simulink model "Explorer1632_LCD"  (Simulink 7.5)
settings: Solver=FixedStepDiscrete  StartTime=0.0  StopTime=200  FixedStep=0.001  RelTol=1e-3
undefined symbols (not defined in the file or in its folder): A0, B15, D4, Max, ms, Pin, Resol, us
libraries: MCHP_Blockset x17, simulink x5
settings Model: Creator=M17129  LastModifiedBy=Lubin Kerhuel
settings OptimizationCC: InlineParams=on  InlineInvariantSignals=on  EnhancedBackFolding=on  ExpressionDepthLimit=128  EfficientFloat2IntCast=on  OptimizeModelRefInitCode=on  LifeSpan=1
settings DebuggingCC: UnderspecifiedInitializationDetection=Simplified  MergeDetectMultiDrivingBlocksExec=error  SolverPrmCheckMsg=none  FcnCallInpInsideContextMsg=Enable All  StateNameClashWarn=none
settings HardwareCC: ProdBitPerInt=16  ProdIntDivRoundTo=Zero  ProdEndianess=LittleEndian  ProdWordSize=16  ProdHWDeviceType=Generic->Custom
settings ModelReferenceCC: ModelReferenceNumInstancesAllowed=Single
settings RTWCC: SystemTargetFile=MCHP_dsPIC_stf.tlc  TemplateMakefile=MCHP_dsPIC.tmf  Description=Microchip Embedded Target PIC24 dsPIC30 dsPIC33 (real-time)  GenerateReport=on  ProcessScript=MCHP_dsPIC_stf_make_rtw_hook  CustomInclude=./clib  CustomSource=Explorer1332_LCD_customCFile.c  IncludeHyperlinkInReport=on  GenerateTraceInfo=on  GenerateTraceReport=on  GenerateTraceReportSl=on  GenerateTraceReportSf=on  GenerateTraceReportEml=on
settings CodeAppCC: ForceParamTrailComments=on  IgnoreCustomStorageClasses=off  MaxIdLength=255  SimulinkDataObjDesc=on  SFDataObjDesc=on  CustomSymbolStrType=$N$R$M_T  InsertBlockDesc=on
settings STFCustomTargetCC: TargetLibSuffix=_lib.a  TargetFunctionLibrary=C89/C90 (ANSI)  IncludeMdlTerminateFcn=off  CombineOutputUpdateFcns=on  SuppressErrorStatus=on  ERTCustomFileBanners=on  SupportContinuousTime=off  SystemTargetFile=MCHP_dsPIC_stf.tlc
settings ERTTargetCC: TargetLibSuffix=_lib.a  TargetFunctionLibrary=C89/C90 (ANSI)  MultiwordLength=2048  ParMdlRefBuildCompliant=off  CompOptLevelCompliant=off  IncludeMdlTerminateFcn=off  SuppressErrorStatus=on  ERTFirstTimeCompliant=off  SupportNonInlinedSFcns=on  ModelStepFunctionPrototypeControlCompliant=off  CPPClassGenCompliant=off  ExtModeMexFile=ext_serial_win32_comm_no_acks  InlinedParameterPlacement=NonHierarchical  ERTSrcFileBannerTemplate=MCHP_dsPIC_code_template.cgt  ERTHdrFileBannerTemplate=MCHP_dsPIC_code_template.cgt  ERTDataSrcFileTemplate=MCHP_dsPIC_code_template.cgt  ERTDataHdrFileTemplate=MCHP_dsPIC_code_template.cgt  ERTCustomFileTemplate=MCHP_main.tlc
settings CustomProperty: DataType=string  Value=33EP512MU810
settings EnumStrPairs: String=elf

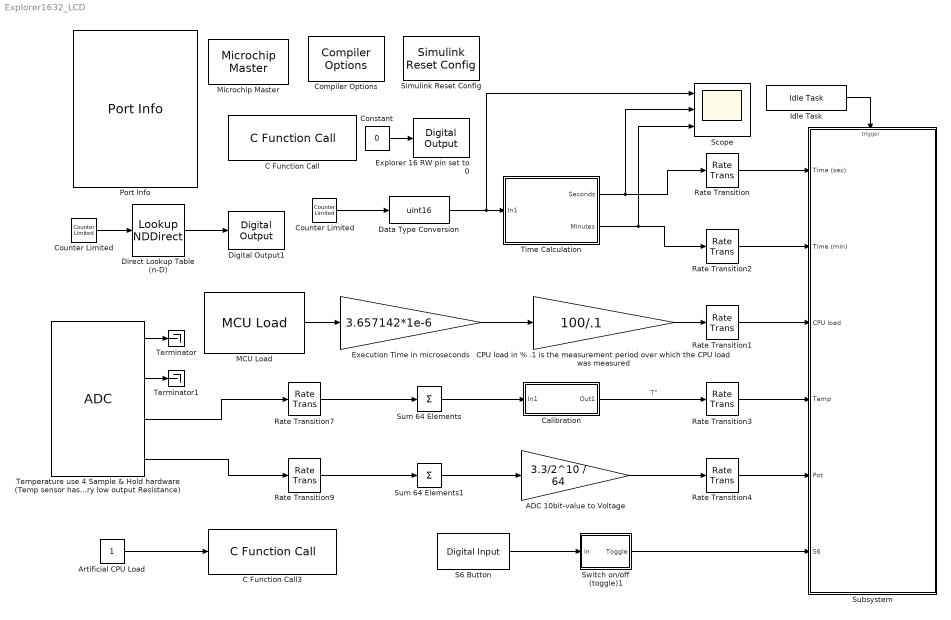
== system Explorer1632_LCD ==
  ADC 10bit-value to Voltage : Gain  Gain=3.3/2^10 / 64  OutDataTypeMode=double  OutDataTypeStr=double
  Artificial CPU Load : Constant  OutDataTypeStr=Inherit: Inherit via back propagation
  C Function Call : MCHP_Blockset/User Functions/C Function Call  ParseFilesChkbx=on  ListFunctions1=Custom Function  Function1=void LCD_StartUp()  AddHeaderDeclaration=off  Function1Type=only once at power-up time  FctReturnBlockOut=off  DataCollected="s.chksm={ '168203-Apr-2017 17:13:43'};s.File1=reshape({ '  void  LCD_StartUp()','  void  PrintMinutes(unsigned int minutes)','  void  PrintSeconds(unsigned int seconds)','  void  PrintVoltage(double v)','  void  PrintTemperature(double temp)','  void  PrintCPU(double CPU_Load)'},1,6);"  ORDERING=None  SampleTime=1  S_INPUT=[]  S_INPUT_Size=[]  S_OUTPUT=[]  S_OUTPUT_Size=[]  S_ListCustomDatatype=S.S_ListCustomDatatype={};  MCHP_CRC=1481661  MCHP_MASTERLINK=Explorer1632_LCD/Microchip Master  PinDigitalInput=[]  PinDigitalOutput=[B15 D4 E[4:7]]  PinAnalogInput=[]  MCHP_PORT={C Function LCD_StartUp}{CFct}10:1:B15;{C Function LCD_StartUp}{CFct}10:1:D4;{C Function LCD_StartUp}{CFct}10:1:E4;{C Function LCD_StartUp}{CFct}10:1:E5;{C Function LCD_StartUp}{CFct}10:1:E6;{C Function LCD_StartUp}{CFct}10:1:E7;
  C Function Call3 : MCHP_Blockset/User Functions/C Function Call  ParseFilesChkbx=off  ListFunctions1=Custom Function  Function1=extern void __delay_us(unsigned long t_us);  AddHeaderDeclaration=off  Function1Type=when block is updated (default)  Fct1BlockIn=t_us  FctReturnBlockOut=off  DataCollected=0  ORDERING=None  SampleTime=.001  S_INPUT=[7]  S_INPUT_Size="[0  0  0  0  0  0  0  0  0  0]"  S_OUTPUT=[]  S_OUTPUT_Size=[]  S_ListCustomDatatype=S.S_ListCustomDatatype={};  MCHP_CRC=972831  MCHP_MASTERLINK=Explorer1632_LCD/Microchip Master  PinDigitalInput=[]  PinDigitalOutput=[]  PinAnalogInput=[]
  CPU load in % .1 is the measurement period over which the CPU load was measured : Gain  Gain=100/.1  ParamDataTypeStr=Inherit: Inherit from 'Gain'  OutDataTypeMode=double  OutDataTypeStr=double
  "Calibration " : Subsystem
  Compiler Options : MCHP_Blockset/System Configuration/Compiler Options  Priority=1  LATEST_CMPLR=on  COMP_LIST=Dynamic Options  COMP_LIST_TXT=xc16 - v1.36  USE_64BIT_DOUBLE=off  MCHP_MULTITHREAD_COMPILATION=on  UseCustom_LinkerScript=off  MCHP_MASTERLINK=Explorer1632_LCD/Microchip Master  OPTIMIZATION_LEVEL=1  OPTIMIZATION_FLTO=on  OPTIMIZATION_REORDER=off  UNROLL_LOOPS=on  PROCEDURAL_ABSTRACTION=off  MPLAB_LINKLIB=default  MPLAB_LINKLIB1=default  MCODE=is less than 32768 (faster)  MCONST=in data memory  MDATA=Use only memory below address 8192 (faster)  MSCALAR=Use only memory below address 8192 (faster)  MLARGEARRAY=off  MAGGREGATE=off  HEAP_SIZE=0  OMF=elf  DEBUG_INFO=off  ProduceHexOutput=off  AssemblyListing=off  NO_EDS_WARN=on  PRINT_STATISTICS=off
  Constant : Constant  Value=0  OutDataType=fixdt(1, 16)  OutScaling=2^0  OutDataTypeStr=Inherit: Inherit via back propagation
  Counter Limited : simulink/Sources/Counter Limited  SystemSampleTime=-1  uplimit=59  tsamp=1
  "Counter Limited " : simulink/Sources/Counter Limited  SystemSampleTime=-1  uplimit=11  tsamp=.08
  Data Type Conversion : DataTypeConversion  OutDataTypeMode=uint16  OutDataTypeStr=uint16  ConvertRealWorld=Stored Integer (SI)
  Digital Output1 : MCHP_Blockset/Digital IO/Digital Output  SystemSampleTime=-1  PORT=Dynamic Options  PORT_TXT="A   [ 0  1  2  3  4  5  6  7  9  10  14  15 ]"  PIN=[1:7]  PACK=on  SIMULTANEOUS=off  READPREVIOUS=off  ORDERING=None  SampleTime=-1  MCHP_MASTERLINK=Explorer1632_LCD/Microchip Master
  Direct Lookup Table (n-D) : LookupNDDirect  NumberOfTableDimensions=1  Table=[ 2 4 8 16 32 64 128 64 32 16 8 4 ]  TableDataTypeStr=uint16
  Execution Time in microseconds : Gain  Gain=3.657142*1e-6  ParamDataTypeStr=Inherit: Inherit from 'Gain'  OutDataTypeMode=double  OutDataTypeStr=double
  Explorer 16 RW pin set to 0 : MCHP_Blockset/Digital IO/Digital Output  SystemSampleTime=-1  PORT=Dynamic Options  PORT_TXT="D   [ 0 : 15 ]"  PIN=5  PACK=off  SIMULTANEOUS=off  READPREVIOUS=off  ORDERING=None  SampleTime=inf  MCHP_MASTERLINK=Explorer1632_LCD/Microchip Master
  Idle Task : MCHP_Blockset/System Functions/Idle Task  MCHP_MASTERLINK=Explorer1632_LCD/Microchip Master
  MCU Load : MCHP_Blockset/Profiling/MCU Load  MCULoadPin=Dynamic Options  MCULoadPin_TXT=None  MCULoadMeasure=on  TIMER_Resolution=Dynamic Options  TIMER_Resolution_TXT="Resol: 3.657(us)  -  Max: 240(ms)"  MCHP_TIMER_REQUEST={MCU_Load}{MCU_Load}21:5:0:0:[]:16777216;  MCHP_TIMER_RESULT=[1 65535 ]  MCHP_MASTERLINK=Explorer1632_LCD/Microchip Master  MCHP_COMPILED_INFO="CompiledSampleTime= [0.10000000000000001   0 ];CompiledInportDataTypes=[ ];CompiledInportDataWidth=[];"  Info="Timer 1:  Resol: 3.657142857(us)  -  Max: 239.675(ms)"  SampleTime=.1
  Microchip Master : MCHP_Blockset/System Configuration/Microchip Master  Priority=1  PICREF=33EP512MU810  TIMESTEP_REF="ADC  ( 0.001s + [0.11429%] ==> 0.0010011s )"  BUSYFLAG=Dynamic Options  BUSYFLAG_TXT=A0 / Pin[17]  PWRTEN=Not used  BOREN=Disable  BODENV=2.7V  BORV=Not used  FPWRT=128ms  DSBOREN=Enable ZPBOR during Deep Sleep Mode  DSLPBOR=Not used  MCLRE=Enabled  SMCLR=MCLR pin generates a normal system Reset  PMDL1WAY=Allow only one reconfiguration  RSTPRI=Device will obtain reset instruction from Primary flash  TEMP=Not used  SOSCSRC=Not used  SOSCSEL=Not used  IOL1WAY=Allow only one reconfiguration  ALTVREF=Not used  DISUVREG=Not used  DSSWEN=Not used  LPCFG=Not used  RTCBAT=Not used  VBTBOR=Not used  WUTSEL=Not used  POWERSAVE=off  FNOSC=Primary Oscillator (XT; HS; EC)  FPR=ECIO w/ PLL 16x  FOSFPR=HS3 w/PLL 16x  FOS=Internal Fast RC  FRANGE=High Range  OSCILLATOR_SELECT=Crystal / Ceramic resonator  OSCILLATOR_SELECT_spd=Crystal / Ceramic resonator  QUARTZ=8e+06  QUARTZ_spd=8e+06  POSCGAIN=2x gain setting  POSCBOOST=Boost the kick start of the oscillator  SOSCGAIN=2x gain setting  SOSCBOOST=Boost the kick start of the oscillator  ACTIV_PLL=on  ACTIV_PLL_spd=on  MIPS_DESIRED=70e+06  MIPS_DESIRED_spd=70e+06  FPLLMUL=Not used  FPLLIDIV=8x Divider  POSCFREQ=Not used  POSCMD=XT Crystal Oscillator Mode  POSCMOD=Primary Oscillator Disabled  MIPS=70 * 1e6  ACLKCON=Optimized for PWM resolution & ADC conversion speed  FPLLODIV=32x Divider  PLLKEN=Clock switch to PLL source will wait until the PLL lock signal is valid.  FCKSM=Clock switching is enabled;Fail-safe Clock Monitor is disabled  FCKSMEN=Sw Disabled; Mon Disabled  IESO=Disable  DSWDTPS=1:2^36  FWDTEN=Disable  FWDTWINSZ=Window size is 25%  FWPSA=1:512  FWPSA0=1:128  FWPSB=1:16  WDT=Disable  WDTPOST=1:32768  WDTPRE=1:128  WDTPS=1:32768  WINDIS=Watchdog Timer in Non-Window mode  WWDTEN=Non-Window mode  DSWDTEN=Enable DSWDT during Deep Sleep Mode  DSWDTOSC=Select LPRC as DSWDT Reference clock  FPBDIV=Not used  FSOSCEN=Enable SOSC  LPRCSEL=Not used  OSCIOFCN=Not used  OSCIOFNC=general purpose digital I/O pin  LVRCFG=Not used  PLL_96MHZ=Not used  PLL96MHZ=Not used  PLLDIV=Not used  WDTCLK=Not used  WDTCMX=Not used  WDTWIN=WDT Window is 25% of WDT period  XTCFG=24-32 MHz crystals  XTBST=Boost the kick-start  APL=Aux Flash Code protect is disabled  APLK=Aux Flash Write Protection and Code Protection is Disabled  AWRP=Auxiliary program memory is not write-protected  BSS=No Boot program Flash segment  BWP=Not used  BWRP=Boot Segment may be written  CP=Protection Disabled  EBS=No Boot EEPROM  ESS=No Segment Data EEPROM  GCP=Disable  GSS=General Segment Code protect is Disabled  GSS0=Not used  GSSK=General Segment Write Protection and Code Protection is Disabled  GWRP=General Segment may be written  PWP=Not used  RBS=No Boot RAM  RSS=No Secure RAM  SSS=No Secure Segment  SWRP=Secure segment may be written  WPCFG=Not used  WPDIS=Not used  WPEND=Not used  WPFP=Not used  ICESEL=Communicate on PGEC1/PGED1  ICS=Communicate on PGEC1 and PGED1  JTAGEN=Disable  COE=Not used  RES=Not used  DEBUG=Debugger is disabled  BACKBUG=Not used  BKBUG=Not used  ALTI2C=I2C mapped to SDA1/SCL1 pins  ALTI2C1=SDA1/SCK1 pins are selected as the I/O pins for I2C1  ALTI2C2=SDA2/SCK2 pins are selected as the I/O pins for I2C2  ALTI2C3=I2C3 mapped to SDA3/SCL3 pins  ALTQIO=QEA1; QEB1; INDX1 are selected as inputs to QEI1  ALTSS1=SS1A is selected as the I/O pin for SPI1  CMPPOL0=Hysteresis is applied to falling edge  CMPPOL1=Hysteresis is applied to falling edge  FCANIO=Not used  FETHIO=Default Ethernet I/O  FMIIEN=MII Enabled  FSRSSEL=Not used  FUSBIDIO=Controlled by the USB Module  FVBUSONIO=Not used  HPOL=Active High  HYST0=45 mV Hysteresis  HYST1=45 mV Hysteresis  I2C1SEL=Not used  LPOL=Active High  PWMPIN=Control with PORT/TRIS regs  RTCOSC=Not used  UPLLEN=USB PLL Disabled  UPLLIDIV=Not used  ATMOD8=Not used  ALTPMP=Not used  I2C2SEL=Not used  ALTADREF=Not used  ALTCVREF=Not used  PWMLOCK=PWM registers may be written without key sequence  INT_PRIORITY_DMA=0  MCHP_TIMER_RESULT=[ ]  MCHP_PORT={Busy Flag}{Busy}0:1:A0;  MCHP_PLLRegisters="[5    243  16385     -1     -1]"  MCHPVAR=MCHP.fcy.MIPS=70000000;MCHP.fcy.SYSCLK=70000000;MCHP.fcy.ADC=70000000;MCHP.fcy.Comparator=70000000;MCHP.fcy.I2C=70000000;MCHP.fcy.SPI=70000000;MCHP.fcy.UART=70000000;MCHP.fcy.Timers=70000000;MCHP.fcy.OC=70000000;MCHP.fcy.IC=70000000;MCHP.fcy.Ports=70000000;MCHP.fcy.QEI=70000000;MCHP.PowerSave=0;MCHP.TimeStepFactor=MCHP_Fun.Hex2num('3FF004AE5F60D755');MCHP.TimeStep_Timer=-1;MCHP.NTIMERS=9;MCHP.id.name='33EP512MU810';MCHP.id.N=reshape([33 512 810],1,3);MCHP.id.L=reshape({ 'EP','MU',''},1,3);MCHP.id.Arch=3;MCHP.periph.PPS.reg_RPINRx=reshape([-1 1 1 1 1 -1 1 1 1 1 1 1 1 1 1 1 1 1 1 1 1 1 -1 -1 1 1 1 1 1 1 1 1 1 1 1 1 1 1 1 1 1 1 1 -1 -1 -1 1 -1 -1 -1 -1 -1 1 1 1 1 1 1 1 1 1 -1 1 1 1 -1 1 1 1 1 1 1 1 1 -1 1 1 1 1 1 1 1 1 -1 1 1 1],1,87);MCHP.PPS.dsPIC.RP=reshape([-1 -1 -1 -1 -1 -1 -1 -1 -1 -1 -1 -1 -1 -1 -1 -1 -1 -1 -1 -1 -1 -1 -1 -1 -1 -1 -1 -1 -1 -1 -1 -1 -1 -1 -1 -1 -1 -1 -1 -1 -1 -1 -1 -1 -1 -1 -1 -1 -1 -1 -1 -1 -1 -1 -1 -1 -1 -1 -1 -1 -1 -1 -1 -1 48 49 50 51 52 53 54 55 -1 -1 -1 -1 -1 -1 -1 63 64 -1 66 -1 68 69 -1 71 -1 -1 -1 -1 -1 -1 -1 -1 80 81 82 83 84 85 -1 -1 88 -1 -1 -1 92 93 -1 -1 96 97 -1 -1 -1 -1 102 -1 104 -1 -1 -1 -1 109 110 111],1,128);MCHP.PPS.dsPIC.RPI=reshape([-1 -1 -1 -1 -1 -1 -1 -1 -1 -1 -1 -1 -1 -1 -1 -1 0 1 2 3 4 5 6 7 -1 -1 -1 -1 -1 -1 14 15 16 17 18 19 20 21 22 23 24 25 26 27 28 29 30 31 -1 33 34 35 36 -1 -1 -1 -1 -1 -1 -1 44 45 46 -1 -1 -1 -1 -1 -1 -1 -1 -1 56 57 58 59 60 61 62 -1 -1 65 -1 67 -1 -1 70 -1 72 73 -1 -1 -1 -1 -1 -1 -1 -1 -1 -1 -1 -1 -1 -1 -1 -1 -1 -1 -1 -1 -1 -1 -1 -1 -1 -1 -1 -1 -1 103 -1 105 -1 -1 108],1,125);MCHP.PPS.dsPIC.RPINR_list=reshape({ '1','INT1','INT2','INT3','INT4','T1CK','T2CK','T3CK','T4CK','T5CK','T6CK','T7CK','T8CK','T9CK','IC1','IC2','IC3','IC4','IC5','IC6','IC7','IC8','OCFA','OCFB','FLT1','FLT2','FLT3','FLT4','QEIA1','QEIB1','QEINDX1','QEIHOM1','QEIA2','QEIB2','QEINDX2','QEIHOM2','U1RX','U1CTS','U2RX','U2CTS','SDI1','SCK1_in','SS1_in','44','SDI2','SCK2_in','SS2_in','48','CSDIR','CSCK','COFS','52','C1RX','C2RX','U3RX','U3CTS','U4RX','U4CTS','SDI3','SCK3_in','SS3_in','62','SDI4','SCK4_in','SS4_in','66','IC9','IC10','IC11','IC12','IC13','IC14','IC15','IC16','OCFC','SYNCI1','SYNCI2','DTCMP1','DTCMP2','DTCMP3','DTCMP4','DTCMP5','DTCMP6','DTCMP7','FLT5','FLT6','FLT7','FLT8','89','SENT1','SENT2','92'},1,92);MCHP.PPS.dsPIC.RPOR_list=reshape({ '1','U1TX','U1RTS','U2TX','U2RTS','SDO1','SCK1_out','SS1_out','SDO2','SCK2_out','SS2_out','CSDO','CSCK','COFS','C1TX','C2TX','OC1','OC2','OC3','OC4','OC5','OC6','OC7','OC8','C1OUT','C2OUT','C3OUT','U3TX','U3RTS','U4TX','U4RTS','SDO3','SCK3_out','SS3_out','SDO4','SCK4_out','SS4_out','OC9','OC10','OC11','OC12','OC13','OC14','OC15','OC16','SYNCO1','SYNCO2','QEI1CCMP','QEI2CCMP','REFCLK','C4OUT','C5OUT','52','53','54','55','56','SENT1','SENT2'},1,59);MCHP.PPS.map_RPnR_RPORx=reshape([64 65 66 67 68 69 70 71 79 80 82 84 85 87 96 97 98 99 100 101 -1 -1 104 108 109 112 113 118 120 125 126 127],1,32);MCHP.Rx=reshape([17 25 -1 72 93 87 90 -1 -1 -1 -1 38 24 6 76 94 88 89 -1 -1 -1 -1 58 23 7 77 98 52 57 -1 -1 -1 -1 59 22 8 78 99 51 56 -1 -1 -1 -1 60 21 9 81 100 49 -1 -1 -1 -1 -1 61 20 -1 82 3 50 -1 -1 -1 -1 -1 91 26 -1 83 4 -1 10 -1 -1 -1 -1 92 27 -1 84 5 -1 11 -1 -1 -1 -1 -1 32 -1 68 18 53 12 -1 -1 -1 -1 28 33 -1 69 19 -1 14 -1 -1 -1 -1 29 34 -1 70 -1 -1 -1 -1 -1 -1 -1 -1 35 -1 71 -1 -1 -1 -1 -1 -1 -1 -1 41 63 79 -1 40 96 -1 -1 -1 -1 -1 42 73 80 -1 39 97 -1 -1 -1 -1 66 43 74 47 -1 -1 95 -1 -1 -1 -1 67 44 64 48 -1 -1 1 -1 -1 -1 -1],11,16);MCHP.ADC.ANtype=reshape([3 1],1,2);MCHP.ADC.ADCONx=reshape([47103 59391 40959 263 0 0],1,6);MCHP.ADC.ADCHS_0=reshape([40863 1799],1,2);MCHP.ADC.Flags=reshape([1 0],1,2);MCHP.ADC.Buffer=reshape([16 16],1,2);MCHP.ADC.port=reshape([16 17 18 19 20 21 22 23 24 25 26 27 28 29 30 31 33 34 35 36 72 73 6 7 64 65 66 67 68 69 70 71 -1 -1 -1 -1 -1 -1 -1 -1 -1 -1 -1 -1 -1 -1 -1 -1 -1 -1 -1 -1 -1 -1 -1 -1 -1],1,57);MCHP.ADC.port_ALT=reshape([-1 -1 -1 -1],1,4);MCHP.ADC.port_VrefP=10;MCHP.ADC.port_VrefM=9;MCHP.ADC.port_AVdd=-1;MCHP.ADC.port_AVss=-1;MCHP.ADC.ADCDATA=reshape([0 0 0 0 0 0 0 0 0 0 0 0 0 0 0 0 0 0 0 0 0 0 0 0 0 0 0 0 0 0 0 0 0 0 0 0 0 0 0 0 0 0 0 0 0 0 0 0 0 0 0 0 0 0 0 0 0],1,57);MCHP.ADC.HS_SAR.TRGSRC=reshape([0 0 0 0 0 0 0 0 0 0 0 0 0 0 0 0 0 0 0 0 0 0 0 0 0 0],1,26);MCHP.ADC.HS_SAR.nFilters=0;MCHP.ADC.HS_SAR.nDedicatedCore=0;MCHP.ADC.HS_SAR.CALIBRATION=0;MCHP.ADC.HS_SAR.ADCON1L=-1;MCHP.memory.RAM=53248;MCHP.memory.RAM_XBegin=4096;MCHP.memory.RAM_YBegin=36864;MCHP.memory.RAM_dma=reshape([53248 57344],1,2);MCHP.memory.FLASH_ECC=0;MCHP.DMA.Num=15;MCHP.DMA.CNTmax=16383;MCHP.QEI.QEICONx=reshape([49023 49023 -1 -1 -1 -1],1,6);MCHP.QEI.QEItype=2;MCHP.QEI.Port_QEI_INDX=reshape([-1 -1],1,2);MCHP.QEI.Port_QEI_QEA=reshape([-1 -1],1,2);MCHP.QEI.Port_QEI_QEB=reshape([-1 -1],1,2);MCHP.QEI.Port_QEI_UPDN=reshape([-1 -1],1,2);MCHP.INT.Port=reshape([48 32767 32767 32767 32767],1,5);MCHP.PWM_HS.Flags=reshape([6 2 1],1,3);MCHP.PWM.port_FLT=reshape([-1 -1 -1 -1 -1 -1 -1 -1 -1 -1 -1 -1 -1 -1 -1 -1 -1 -1 -1 -1 -1 -1 -1 -1 -1 -1 -1 -1 -1 -1 -1 -1 -1],1,33);MCHP.PWM.PWMRef=-1;MCHP.PWM.Flag=0;MCHP.PWM.Port_PWM_l=reshape([64 -1 66 -1 68 -1 70 -1 33 -1 35 -1 -1 -1 -1 -1 -1 -1 -1 -1 -1 -1 -1 -1],2,12);MCHP.PWM.Port_PWM_h=reshape([65 -1 67 -1 69 -1 71 -1 34 -1 36 -1 -1 -1 -1 -1 -1 -1 -1 -1 -1 -1 -1 -1],2,12);MCHP.PWM_HS_FEP.nEVTOUT=-1;MCHP.IC.Port=reshape([32767 32767 32767 32767 32767 32767 32767 32767 32767 32767 32767 32767 32767 32767 32767 32767],1,16);MCHP.IC.type=1;MCHP.OC.Port=reshape([32767 32767 32767 32767 32767 32767 32767 32767 32767 32767 32767 32767 32767 32767 32767 32767],1,16);MCHP.OC.type=1;MCHP.CN.Port=reshape([-1 -1 -1 -1 -1 -1 -1 -1 -1 -1 -1 -1 -1 -1 -1 -1 -1 -1 -1 -1 -1 -1 -1 -1 -1 -1 -1 -1 -1 -1 -1 -1 -1 -1 -1 -1 -1 -1 -1 -1 -1 -1 -1 -1 -1 -1 -1 -1 -1 -1 -1 -1 -1 -1 -1 -1 -1 -1 -1 -1 -1 -1 -1 -1 -1 -1 -1 -1 -1 -1 -1 -1 -1 -1 -1 -1 -1 -1 -1 -1 -1 -1 -1 -1 -1],1,85);MCHP.CN.PullUp=reshape([50943 65535 61470 65535 1023 12607 62403 0 0 0 0],1,11);MCHP.CN.type=1;MCHP.CN.Flag_PullDown=1;MCHP.SPI.Refs=reshape([1 2 3 4 0 0],1,6);MCHP.SPI.SPIxCON1=8191;MCHP.SPI.SPIxCON2=57347;MCHP.SPI.Port_SDI=reshape([-1 103 -1 -1 -1 -1],1,6);MCHP.SPI.Port_SDO=reshape([-1 104 -1 -1 -1 -1],1,6);MCHP.SPI.Port_SCK=reshape([-1 102 -1 -1 -1 -1],1,6);MCHP.SPI.Port_SS=reshape([-1 -1 -1 -1 -1 -1],1,6);MCHP.I2C.Refs=reshape([1 2 0 0 0],1,5);MCHP.I2C.I2CxCON=49151;MCHP.I2C.NewRegName=1;MCHP.I2C.Port_SDA=reshape([-1 84 -1 -1 -1],1,5);MCHP.I2C.Port_SCL=reshape([-1 85 -1 -1 -1],1,5);MCHP.I2C.Port_ASDA=reshape([57 3 -1 -1 -1],1,5);MCHP.I2C.Port_ASCL=reshape([58 2 -1 -1 -1],1,5);MCHP.I2C.Fuse_Port_SCL_SDA=reshape([17 1 18 1 -1 -1 -1 -1 -1 -1],2,5);MCHP.I2C.Fuse_Port_ASCL_ASDA=reshape([17 2 18 2 -1 -1 -1 -1 -1 -1],2,5);MCHP.SCCP.nSCCP=0;MCHP.SCCP.MCCP=reshape([0 0 0 0 0 0 0 0 0],1,9);MCHP.PGA.Port_PGA1P=reshape([-1 -1 -1 -1],1,4);MCHP.PGA.Port_PGA1N=reshape([-1 -1 -1 -1],1,4);MCHP.PGA.Port_PGA2P=reshape([-1 -1 -1 -1],1,4);MCHP.PGA.Port_PGA2N=reshape([-1 -1 -1 -1],1,4);MCHP.PGA.Num=0;MCHP.HS_AnalogComparator.Port_CMP1=reshape([-1 -1 -1 -1],1,4);MCHP.HS_AnalogComparator.Port_CMP2=reshape([-1 -1 -1 -1],1,4);MCHP.HS_AnalogComparator.Port_CMP3=reshape([-1 -1 -1 -1],1,4);MCHP.HS_AnalogComparator.Port_CMP4=reshape([-1 -1 -1 -1],1,4);MCHP.HS_AnalogComparator.PORT_EXTREFx=reshape([-1 -1],1,2);MCHP.HS_AnalogComparator.Port_DACOUTx=reshape([-1 -1],1,2);MCHP.HS_AnalogComparator.Num=0;MCHP.Comp.Port_CVrefin=-1;MCHP.Comp.Port_CVref=26;MCHP.Comp.Port_CVref1O=-1;MCHP.Comp.Port_CVref2O=-1;MCHP.Comp.Port_CxOUT=reshape([32767 32767 32767 -1 -1],1,5);MCHP.Comp.Port_OAxOUT=reshape([-1 -1 -1 -1 -1],1,5);MCHP.Comp.Port_CxINP=reshape([21 19 55 -1 -1],1,5);MCHP.Comp.Port_CxINM=reshape([103 20 102 -1 105 18 104 -1 46 54 45 -1 -1 -1 -1 -1 -1 -1 -1 -1],4,5);MCHP.Comp.Port_OAxINP=reshape([-1 -1 -1 -1 -1],1,5);MCHP.Comp.Port_OAxINM=reshape([-1 -1 -1 -1 -1],1,5);MCHP.Comp.nComp=reshape([3 0 0],1,3);MCHP.Comp.OpAmp=0;MCHP.Comp.CVRCON=reshape([2047 0],1,2);MCHP.CDAC.Port_DACx=reshape([-1 -1 -1],1,3);MCHP.CDAC.nCDAC=0;MCHP.UART.port_Rx=reshape([32767 32767 32767 32767 -1 -1],1,6);MCHP.UART.port_Tx=reshape([32767 32767 32767 32767 -1 -1],1,6);MCHP.UART.port_ARx=reshape([-1 -1],1,2);MCHP.UART.port_ATx=reshape([-1 -1],1,2);MCHP.UART.port_RTS=reshape([32767 32767 32767 32767 -1 -1],1,6);MCHP.UART.port_CTS=reshape([32767 32767 32767 32767 -1 -1],1,6);MCHP.UART.reg_UxMODE=reshape([48127 48127 48127 48127 -1 -1],1,6);MCHP.UART.reg_UxSTA=reshape([61439 61439 61439 61439 -1 -1],1,6);MCHP.modsrc.DOS_02551_cpu_16bit_v7=0;MCHP.modsrc.DOS_01520_wdt_dmt_upb_v1_16bit=0;MCHP.modsrc.DOS_02359a_sent_j2716_upb_v1=0;MCHP.modsrc.DOS_02672_math_progcrc_upb_v1_16bit=0;MCHP.modsrc.DOS_01577_cla_clc_upb_v1=0;MCHP.modsrc.DOS_02915_ecc_v2=0;MCHP.modsrc.DOS_02673_tmr_classa_upb_v1_16bit=0;MCHP.modsrc.DOS_01494_qei_32b_upb_v1_16bit=0;MCHP.modsrc.DOS_02552_msi_upb_v1_Master=0;MCHP.modsrc.DOS_01441_i2c_upb_v1_16bit_TLAH=0;MCHP.modsrc.DOS_03076_uart_protocol_upb_v1_16bit=0;MCHP.modsrc.DOS_01482=0;MCHP.modsrc.DOS_01483_pwm_16bit=0;MCHP.modsrc.DOS_03247_CAN_FD_UPB_V2_16_bit=0;MCHP.modsrc.DOS_02497_WACV=0;MCHP.modsrc.DOS_02316_nvm_ctrl_v1_16bit=0;MCHP.modsrc.DOS_02653_afe_current_bias_ctrl_upb_v1_16bit=0;MCHP.modsrc.DOS_01459_ptg_pc_upb_v1_16bit=0;MCHP.modsrc.DOS_01512_ccp_mccp_upb_v1_16bit=0;MCHP.modsrc.DOS_02519_dma_sfr_16bit_v2=0;MCHP.modsrc.DOS_02508c11=0;MCHP.modsrc.DOS_02475_dac_pdm_nbit_upb_v1_16bit=0;MCHP.modsrc.DOS_02467_gpio_upb_v1_16bit=0;MCHP.modsrc.DOS_00805_rst_integration_v4=0;MCHP.modsrc.DOS_02659_clk_sib_v12=0;MCHP.modsrc.DOS_02674_wdt_upb_v1_16bit=0;MCHP.modsrc.DOS_01407=0;MCHP.modsrc.DOS_02552_msi_upb_v1_Slave=0;MCHP.modsrc.DOS_02593_amp_pga_ctrl_pb_v2_16bit=0;MCHP.modsrc.DOS_01461_afe_ctmu_con_upb_v1_16bit=0;MCHP.modsrc.DOS_02497_WACA=0;MCHP.modsrc.DOS_02478_uart_irda_upb_v1_16bit=0;MCHP.modsrc.DOS_00929=1;MCHP.modsrc.DOS_01198=1;MCHP.modsrc.DOS_03029_WACH=0;MCHP.modsrc.DOS_02472_ppi_pmp16_upb_v1_16bit=0;MCHP.modsrc.DOS_02949_WACG=0;MCHP.modsrc.DOS_03349_amp_pad_opamp_ctrl_upb_v1=0;MCHP.modsrc.DOS_02237_osc_dco_ctrl_upb_v1_16bit=0;MCHP.modsrc.DOS_03662_WACU=0;MCHP.modsrc.DOS_03994_WAC07_Module=0;MCHP.modsrc.DOS_00794=1;MCHP.modsrc.DOS_00931=1;MCHP.modsrc.DOS_00932=1;MCHP.modsrc.DOS_00942=1;MCHP.modsrc.DOS_00938=1;MCHP.modsrc.DOS_00996=1;MCHP.modsrc.DOS_00997=1;MCHP.modsrc.DOS_00998=1;MCHP.modsrc.DOS_00209=1;MCHP.modsrc.DOS_01555_adc=0;MCHP.modsrc.DOS_01293=0;MCHP.modsrc.DOS_00828=1;MCHP.modsrc.DOS_01116=1;MCHP.modsrc.DOS_01017_RPORx=1;MCHP.modsrc.DOS_01017_RPINRx=1;MCHP.modsrc.DOS_01555_nvm_tsmc18_v2_16bit=0;MCHP.modsrc.DOS_00804=1;MCHP.modsrc.DOS_00826=1;MCHP.modsrc.DOS_01555_TLAK_PMDx=0;MCHP.modsrc.DOS_01555_TLAK_INT_=0;MCHP.modsrc.DOS_00933=1;MCHP.modsrc.DOS_01555=0;MCHP.modsrc.DOS_01555_ptg=0;MCHP.modsrc.DOS_00958=1;MCHP.modsrc.DOS_01117_PORTx=1;MCHP.modsrc.DOS_00999=1;MCHP.modsrc.DOS_01041=1;MCHP.modsrc.DOS_00892=1;MCHP.modsrc.DOS_01287_TLAC_PMDx=0;MCHP.modsrc.DOS_01287_TLAC_INT_=0;MCHP.modsrc.DOS_01424=0;MCHP.modsrc.DOS_01332=0;MCHP.modsrc.DOS_01468_PMBA_current_source=0;MCHP.modsrc.DOS_02291_PGA=0;MCHP.modsrc.DOS_01467_Comparator=0;MCHP.modsrc.DOS_01498_TLAY=0;MCHP.modsrc.DOS_00993_PLL_120MHz=0;MCHP.modsrc.DOS_01332_ptg_pc_v1=0;MCHP.modsrc.DOS_00958_pwm_TLAY=0;MCHP.modsrc.TLAY_IOPorts=0;MCHP.modsrc.DOS_00929q=0;MCHP.modsrc.DOS_02415_spi_v5=0;MCHP.modsrc.DOS_RPINRx_16bit_2=0;MCHP.modsrc.DOS_01497_TLAH_PMDx=0;MCHP.modsrc.DOS_02550_TLAL_INT=0;MCHP.modsrc.DOS_00958_pwm_TLAH=0;MCHP.modsrc.DOS_01287_TLAH_INT_=0;MCHP.modsrc.DOS_01113=1;MCHP.modsrc.DOS_01017_PMDx=1;MCHP.modsrc.DOS_00927=1;MCHP.modsrc.DOS_01080=1;MCHP.modsrc.DOS_00794_cpu_16bit_v3=0;MCHP.modsrc.DOS_02192_TLCD_PMDx=0;MCHP.modsrc.DOS_02192_TLCD_INT_=0;MCHP.modsrc.DOS_02192_cmp=0;MCHP.modsrc.DOS_00958_pwm_TLCD=0;MCHP.modsrc.DOS_02192_PORTx_TLCD=0;MCHP.modsrc.DOS_00936=0;MCHP.modsrc.DOS_00995=0;MCHP.modsrc.DOS_00546=0;MCHP.modsrc.DOS_00474=0;MCHP.modsrc.DOS_02481_WACJ_MC_Config=0;MCHP.modsrc.DOS_02569_pfm_cache_ocp_v1=0;MCHP.modsrc.DOS_02819_pfm_ctrl_32bit_upb_v2=0;MCHP.modsrc.DOS_02674_wdt_upb_v1_32bit=0;MCHP.modsrc.DOS_01520_wdt_dmt_upb_v1=0;MCHP.modsrc.DOS_02869_icd_jtag_bvci_upb_v2=0;MCHP.modsrc.DOS_02823_WACJ_clk_cru_upb_v2=0;MCHP.modsrc.DOS_01423_RPINRx=0;MCHP.modsrc.DOS_02481_RPORx=0;MCHP.modsrc.DOS_02511_pwr_sib_upb_v1_32bit=0;MCHP.modsrc.DOS_02481_WACJ_MC_int_evic_v3=0;MCHP.modsrc.DOS_01500_dma_bvci_v2=0;MCHP.modsrc.DOS_02141_tmr_classa_pb_v2=0;MCHP.modsrc.DOS_02815_tmr_classb_upb_v1=0;MCHP.modsrc.DOS_00740_icap_pb_v1=0;MCHP.modsrc.DOS_00749_ocmp_pb_v1=0;MCHP.modsrc.DOS_01441_i2c_upb_v1_32bit=0;MCHP.modsrc.DOS_01329_spi_pb_v2=0;MCHP.modsrc.DOS_02478_uart_irda_upb_v1_32bit=0;MCHP.modsrc.DOS_02514_dfm_strl_sst_upb_v1=0;MCHP.modsrc.DOS_01477_pwm_mc_upb_v1=0;MCHP.modsrc.DOS_01459_ptg_pc_upb_v1_SIC=0;MCHP.modsrc.DOS_01494_qei_32b_upb_v1=0;MCHP.modsrc.DOS_01427_cmp_control_upb_v1_32bit=0;MCHP.modsrc.DOS_01445_dac_nbit__control_upb_v1_32bit=0;MCHP.modsrc.DOS_01461_afe_ctmu_con_upb_v1=0;MCHP.modsrc.DOS_02472_ppi_pmp16_upb_v1=0;MCHP.modsrc.DOS_02467_gpio_ports_upb_v1=0;MCHP.modsrc.DOS_01152_can_bvci_v1=0;MCHP.modsrc.DOS_02508_adc_sar_ctrl_upb_v1_PIC32MK=0;MCHP.modsrc.DOS_02813a_usb_otgcore_pb_v3=0;MCHP.modsrc.DOS_01261_tmr_rtcc_pb_v2=0;MCHP.modsrc.DOS_01475_lpwr_deep_sleep_ctrl_v2=0;MCHP.modsrc.DOS_EIP_00136_ssx_v1=0;MCHP.modsrc.DOS_02481_WACK_MC_Config=0;MCHP.modsrc.DOS_03088_pfm_cache_ocp_v2_WACK=0;MCHP.modsrc.DOS_02823_WACN_clk_cru_upb_v2=0;MCHP.modsrc.DOS_02907_WACK_MC_int_evic_v3=0;MCHP.modsrc.DOS_03554_cmp_control_upb_v2_32bit=0;MCHP.modsrc.DOS_03247_can_fd_upb_v2_pic32mk=0;MCHP.modsrc.DOS_02787_WACD_Config=0;MCHP.modsrc.DOS_00800_dac_4bit_ctrl_pb_v1=0;MCHP.modsrc.DOS_01539_icd_jtag_pb_v2=0;MCHP.modsrc.DOS_02823_clk_cru_upb_v2=0;MCHP.modsrc.DOS_01423_RPORx=0;MCHP.modsrc.DOS_02907_WACD_int_evic_v3=0;MCHP.modsrc.DOS_00734_uart_irda_pb_v1=0;MCHP.modsrc.DOS_00687_tmr_classa_pb_v1=0;MCHP.modsrc.DOS_00745_tmr_classb_pb_v1=0;MCHP.modsrc.DOS_02508_adc_sar_ctrl_upb_v1=0;MCHP.modsrc.DOS_00866_cmp_control_pb_v2=0;MCHP.modsrc.DOS_01114_eth_bvci_v1=0;MCHP.modsrc.DOS_02831_usb_clk_rst_v2=0;MCHP.modsrc.DOS_01643_pfm_cache_ahb_v2=0;MCHP.modsrc.DOS_EIP_00206r5_sqi_v2=0;MCHP.modsrc.DOS_EIP_00124_usb_hs_otgcore_v1=0;MCHP.modsrc.DOS_EIP_00218_math_rng_ahbs_v2=0;MCHP.modsrc.DOS_EIP_00109_ebi_v1=0;MCHP.modsrc.DOS_EIP_00158_crypto_v1=0;MCHP.PortBase=16;MCHP.PortPrefixe='P';MCHP.clock.PBxDIV=-1;  MCHP_CRC=6245820  BTMODE=Not used  RES1=Not used  PLLSS=Not used  RES2=Not used  ALTCMPI=Not used  BOREN1=Not used  ALTRB6=Not used  RETCFG=Not used  DFMCY=Not used  BSS2=No Boot Segment  BSEN=No Boot Segment  CWRP=Configuration Segment may be written  CSS=No Protection (other than CWRP)  AIVTDIS=Disable Alternate Vector Table  BSLIM=Not used  WDTEN=Disable  BTSWP=BOOTSWP instruction is disabled  DBCC=No Cross Connection between DAC outputs  CTXT1=Not Assigned  CTXT2=Not Assigned  SEQNUM=Not used  nSEQNUM=Not used  BOREN0=Enabled  DMTIVT=Not used  DMTCNT=2^31 (2147483648)  DMTEN=Dead Man Timer is Disabled and can be enabled by software  ON=Not used  USERID=Not used  RESERVED1=Not used  PGL1WAY=Allow only one reconfiguration  FPLLRNG=34-68 MHz Input  FPLLICLK=FRC is input to the System PLL  FPLLMULT=PLL Multiply by 128  UPLLFSEL=USB PLL input is 24 MHz  DMTINTV=Window/Interval value is 127/128 counter value  WDTSPGM=WDT stops during Flash programming  FDMTEN=Deadman Timer is disabled  TRCEN=Trace features in the CPU are enabled  BOOTISA=Boot code and Exception code is MIPS32  FECCCON=ECC and Dynamic ECC are disabled (ECCCON bits are writable)  EXTDDRSIZE=Not used  FSLEEP=Flash is powered down when the device is in Sleep mode  DBGPER=Allow CPU access to all permission regions  EJTAGBEN=Normal EJTAG functionality  TSEQ=Not used  CSEQ=Not used
  Port Info : MCHP_Blockset/System Info/Port Info  MCHP_MASTERLINK=Explorer1632_LCD/Microchip Master
  Rate Transition{,1..4} (5 alike) : RateTransition  Deterministic=off  OutPortSampleTimeOpt=Inherit
  Rate Transition7 : RateTransition  Deterministic=off  OutPortSampleTime=0.2
  Rate Transition9 : RateTransition  Deterministic=off  OutPortSampleTime=[0.2 0.1]
  S6 Button : MCHP_Blockset/Digital IO/Digital Input  PORT=Dynamic Options  PORT_TXT="D   [ 0 : 15 ]"  PIN=13  PACK=off  SIMULTANEOUS=off  ORDERING=None  SampleTime=.01  MCHP_PORT={Digital In}{DIN}2:0:D13;  MCHP_MASTERLINK=Explorer1632_LCD/Microchip Master
  Scope : Scope  NumInputPorts=3
      settings: YMin=-7.375~-4.47906~-0.375  YMax=66.375~62.70681~3.375
  Simulink Reset Config : MCHP_Blockset/System Configuration/Simulink Reset Config  MCHP_MASTERLINK=0
  Subsystem : Subsystem
  Sum 64 Elements : Sum  Inputs=+
  Sum 64 Elements1 : Sum  Inputs=+
  Switch on/off (toggle)1 : Subsystem
  Temperature use 4 Sample & Hold hardware (Temp sensor has very low output Resistance) : MCHP_Blockset/Analog IO/ADC  Priority=5  ADC_REF=1  Mode=10 bits (allows exact simultaneous sampling)  FORM=0000 dddd dddd dddd ==> Unsigned integer  ADC_R="< 1    kOhm"  nSAMPLECHANNELS=CH0 : CH1 : CH2 : CH3  nSAMPLECHANNELS_12bits=CH0 only  SIMULTANEOUS=Simultaneously on all Channels  ADxCSS=[5]  MUXA_CH0N=off  MUXA_CH123=Dynamic Options  MUXA_CH123_TXT=AN3 : AN4 : AN5  MUXB_CH0=AN1  MUXB_CH0N=on  MUXB_CH123=Dynamic Options  MUXB_CH123_TXT=AN0 : AN1 : AN2  SequenceRepeat=64  SequenceTiming=are stretcheded to fit exactly previous time step  SSRC_SSRCG=Dynamic Options  SSRC_SSRCG_TXT=6  Update_BlockOutput=After all trig and conversion sequence  Trig_TimeStep=with each update of the ADC block output  ADC_DMA_CHANNEL=use DMA Channel 0  SampleTime=0.001  Info=Total Time for Sample & Conversion : 0.0010011s including 5.3571e-006s (x 64) sample time. Difference with time step is : 1.1429e-006s  MCHP_PORT={Analog Input 3}{AN3}15:2:B3;{Analog Input 4}{AN4}15:2:B4;{Analog Input 5}{AN5}15:2:B5;  MCHP_MASTERLINK=Explorer1632_LCD/Microchip Master  ADC_TIMING=[0.0010011428571428571]
  Terminator : Terminator
  Terminator1 : Terminator
  Time Calculation : Subsystem  TreatAsAtomicUnit=on
  wires:
  Counter Limited/1 -> Data Type Conversion/1
  Idle Task/1 -> Subsystem/Trigger
  Rate Transition/1 -> Subsystem/1(Time (sec))
  Time Calculation/1(Seconds) -> Scope/2, Rate Transition/1
  Time Calculation/2(Minutes) -> Scope/3, Rate Transition2/1
  Rate Transition2/1 -> Subsystem/2(Time (min))
  Data Type Conversion/1 -> Scope/1, Time Calculation/1(In1)
  "Counter Limited "/1 -> Direct Lookup Table (n-D)/1
  Direct Lookup Table (n-D)/1 -> Digital Output1/1
  Artificial CPU Load/1 -> C Function Call3/1
  Rate Transition9/1 -> Sum 64 Elements1/1
  Temperature use 4 Sample & Hold hardware (Temp sensor has very low output Resistance)/4 -> Rate Transition9/1
  Sum 64 Elements/1 -> "Calibration "/1(In1)
  Execution Time in microseconds/1 -> CPU load in % .1 is the measurement period over which the CPU load was measured/1
  Sum 64 Elements1/1 -> ADC 10bit-value to Voltage/1
  Rate Transition7/1 -> Sum 64 Elements/1
  MCU Load/1 -> Execution Time in microseconds/1
  Rate Transition3/1 -> Subsystem/4(Temp)
  Temperature use 4 Sample & Hold hardware (Temp sensor has very low output Resistance)/3 -> Rate Transition7/1
  "Calibration "/1(Out1) -> Rate Transition3/1  "T°"
  Switch on/off (toggle)1/1(Toggle) -> Subsystem/6(S6)
  S6 Button/1 -> Switch on/off (toggle)1/1(in)
  Rate Transition4/1 -> Subsystem/5(Pot)
  ADC 10bit-value to Voltage/1 -> Rate Transition4/1
  Rate Transition1/1 -> Subsystem/3(CPU load)
  Temperature use 4 Sample & Hold hardware (Temp sensor has very low output Resistance)/1 -> Terminator/1
  Temperature use 4 Sample & Hold hardware (Temp sensor has very low output Resistance)/2 -> Terminator1/1
  CPU load in % .1 is the measurement period over which the CPU load was measured/1 -> Rate Transition1/1
  Constant/1 -> Explorer 16 RW pin set to 0/1

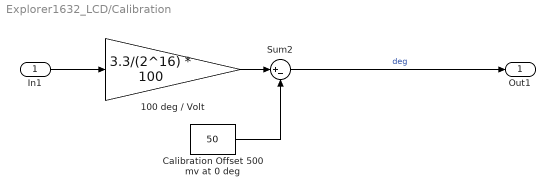
== system Explorer1632_LCD/Calibration  ==
  In1 : Inport
  "100 deg / Volt " : Gain  Gain=3.3/(2^16) * 100  OutDataTypeMode=single  OutDataTypeStr=single
  Calibration Offset 500 mv at 0 deg : Constant  Value=50  OutDataTypeStr=Inherit: Inherit via back propagation  SampleTime=-1
  Sum2 : Sum  Inputs=|+-
  Out1 : Outport
  wires:
  In1/1 -> "100 deg / Volt "/1
  "100 deg / Volt "/1 -> Sum2/1
  Calibration Offset 500 mv at 0 deg/1 -> Sum2/2
  Sum2/1 -> Out1/1  "deg"

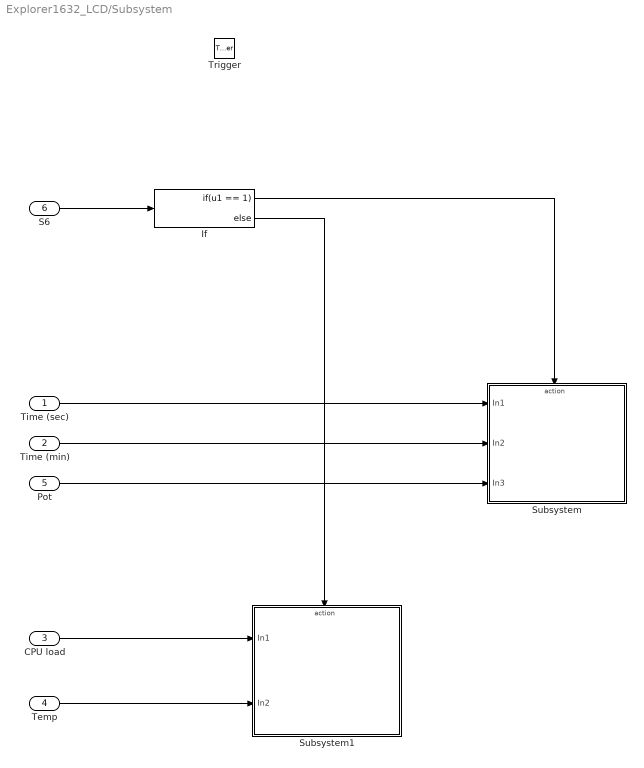
== system Explorer1632_LCD/Subsystem ==
  Time (sec) : Inport
  Time (min) : Inport  Port=2
  CPU load : Inport  Port=3
  Temp : Inport  Port=4
  Pot : Inport  Port=5
  S6 : Inport  Port=6
  Trigger : TriggerPort  TriggerType=function-call  PortDimensions=1
  If : If  IfExpression=u1 == 1
  Subsystem : Subsystem
  Subsystem1 : Subsystem
  wires:
  Time (sec)/1 -> Subsystem/1(In1)
  Time (min)/1 -> Subsystem/2(In2)
  Pot/1 -> Subsystem/3(In3)
  S6/1 -> If/1
  CPU load/1 -> Subsystem1/1(In1)
  Temp/1 -> Subsystem1/2(In2)
  If/1 -> Subsystem/Action
  If/2 -> Subsystem1/Action

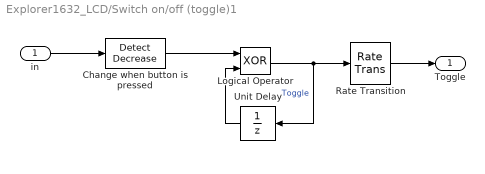
== system Explorer1632_LCD/Switch on/off (toggle)1 ==
  in : Inport
  Change when button is pressed : simulink/Logic and Bit Operations/Detect Decrease  SystemSampleTime=-1  vinit=0.0
  Logical Operator : Logic  Operator=XOR  AllPortsSameDT=off  OutDataTypeMode=boolean  OutDataTypeStr=boolean
  Rate Transition : RateTransition  Integrity=off  Deterministic=off
  Unit Delay : UnitDelay  SampleTime=-1
  Toggle : Outport
  wires:
  Rate Transition/1 -> Toggle/1
  Logical Operator/1 -> Rate Transition/1, Unit Delay/1  "Toggle"
  in/1 -> Change when button is pressed/1
  Change when button is pressed/1 -> Logical Operator/1
  Unit Delay/1 -> Logical Operator/2

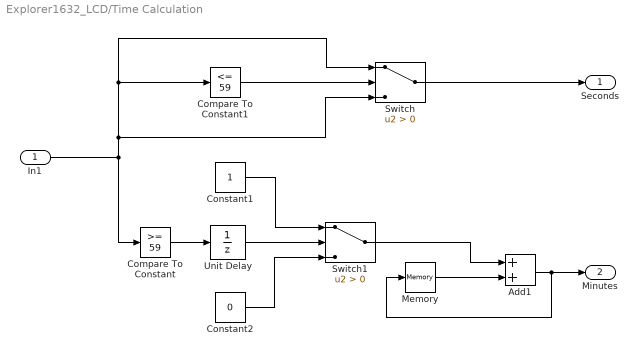
== system Explorer1632_LCD/Time Calculation ==
  In1 : Inport
  Add1 : Sum  AccumDataTypeStr=uint16
  Compare To Constant : simulink/Logic and Bit Operations/Compare To Constant  SystemSampleTime=-1  relop=>=  const=59  LogicOutDataTypeMode=boolean
  Compare To Constant1 : simulink/Logic and Bit Operations/Compare To Constant  SystemSampleTime=-1  relop=<=  const=59  LogicOutDataTypeMode=boolean
  Constant1 : Constant  SampleTime=-1
  Constant2 : Constant  Value=0  OutDataTypeStr=Inherit: Inherit via back propagation  SampleTime=-1
  Memory : Memory  InheritSampleTime=on  LinearizeAsDelay=on
  Switch : Switch  Criteria=u2 > Threshold  OutDataTypeMode=uint16  OutDataTypeStr=uint16
  Switch1 : Switch  Criteria=u2 > Threshold  OutDataTypeMode=uint16  OutDataTypeStr=uint16
  Unit Delay : UnitDelay  SampleTime=-1
  Seconds : Outport
  Minutes : Outport  Port=2
  wires:
  Compare To Constant1/1 -> Switch/2
  Compare To Constant/1 -> Unit Delay/1
  Constant2/1 -> Switch1/3
  Constant1/1 -> Switch1/1
  Switch/1 -> Seconds/1
  Switch1/1 -> Add1/1
  Add1/1 -> Minutes/1, Memory/1
  Memory/1 -> Add1/2
  In1/1 -> Switch/1, Compare To Constant1/1, Switch/3, Compare To Constant/1
  Unit Delay/1 -> Switch1/2

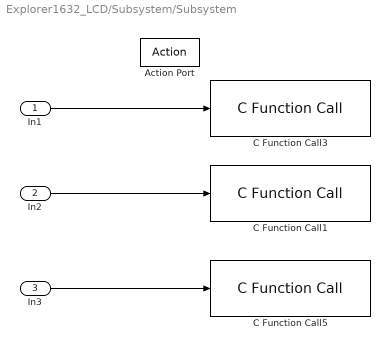
== system Explorer1632_LCD/Subsystem/Subsystem ==
  In1 : Inport
  In2 : Inport  Port=2
  In3 : Inport  Port=3
  Action Port : ActionPort  ActionType=then
  C Function Call1 : MCHP_Blockset/User Functions/C Function Call  ParseFilesChkbx=on  ListFunctions1=Custom Function  Function1=void PrintMinutes(unsigned int value)  AddHeaderDeclaration=on  Function1Type=when block is updated (default)  Fct1BlockIn=minutes  FctReturnBlockOut=off  DataCollected="s.chksm={ '132103-Apr-2017 16:24:15'};s.File1=reshape({ '  void  ShowOff()','  void  PrintMinutes(unsigned int minutes)','  void  PrintSeconds(unsigned int seconds)','  void  PrintVoltage(double v)','  void  PrintCPU(double CPU_Load)','  void  PrintTemperature(double temp)'},1,6);"  ORDERING=None  SampleTime=-1  S_INPUT=[5]  S_INPUT_Size="[0  0  0  0  0  0  0  0  0  0]"  S_OUTPUT=[]  S_OUTPUT_Size=[]  S_ListCustomDatatype=S.S_ListCustomDatatype={};  MCHP_CRC=1289421  MCHP_MASTERLINK=Explorer1632_LCD/Microchip Master  PinDigitalInput=[]  PinDigitalOutput=[]  PinAnalogInput=[]
  C Function Call3 : MCHP_Blockset/User Functions/C Function Call  ParseFilesChkbx=on  ListFunctions1=Custom Function  Function1=void PrintSeconds(unsigned int seconds)  AddHeaderDeclaration=on  Function1Type=when block is updated (default)  Fct1BlockIn=seconds  FctReturnBlockOut=off  DataCollected="s.chksm={ '132103-Apr-2017 16:24:15'};s.File1=reshape({ '  void  ShowOff()','  void  PrintMinutes(unsigned int minutes)','  void  PrintSeconds(unsigned int seconds)','  void  PrintVoltage(double v)','  void  PrintCPU(double CPU_Load)','  void  PrintTemperature(double temp)'},1,6);"  ORDERING=None  SampleTime=-1  S_INPUT=[5]  S_INPUT_Size="[0  0  0  0  0  0  0  0  0  0]"  S_OUTPUT=[]  S_OUTPUT_Size=[]  S_ListCustomDatatype=S.S_ListCustomDatatype={};  MCHP_CRC=1291597  MCHP_MASTERLINK=Explorer1632_LCD/Microchip Master  PinDigitalInput=[]  PinDigitalOutput=[]  PinAnalogInput=[]
  C Function Call5 : MCHP_Blockset/User Functions/C Function Call  ParseFilesChkbx=on  ListFunctions1=Custom Function  Function1=void PrintVoltage(double v)  AddHeaderDeclaration=on  Function1Type=when block is updated (default)  Fct1BlockIn=v  FctReturnBlockOut=off  DataCollected="s.chksm={ '132103-Apr-2017 16:24:15'};s.File1=reshape({ '  void  ShowOff()','  void  PrintMinutes(unsigned int minutes)','  void  PrintSeconds(unsigned int seconds)','  void  PrintVoltage(double v)','  void  PrintCPU(double CPU_Load)','  void  PrintTemperature(double temp)'},1,6);"  ORDERING=None  SampleTime=-1  S_INPUT=[0]  S_INPUT_Size="[0  0  0  0  0  0  0  0  0  0]"  S_OUTPUT=[]  S_OUTPUT_Size=[]  S_ListCustomDatatype=S.S_ListCustomDatatype={};  MCHP_CRC=1223165  MCHP_MASTERLINK=Explorer1632_LCD/Microchip Master  PinDigitalInput=[]  PinDigitalOutput=[]  PinAnalogInput=[]
  wires:
  In3/1 -> C Function Call5/1
  In2/1 -> C Function Call1/1
  In1/1 -> C Function Call3/1

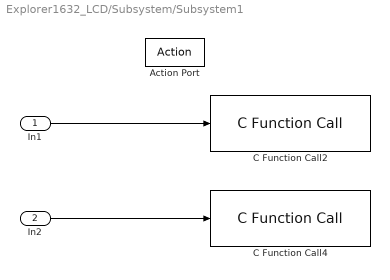
== system Explorer1632_LCD/Subsystem/Subsystem1 ==
  In1 : Inport
  In2 : Inport  Port=2
  Action Port : ActionPort  ActionType=else
  C Function Call2 : MCHP_Blockset/User Functions/C Function Call  ParseFilesChkbx=on  ListFunctions1=Custom Function  Function1=void PrintCPU(double CPU_Load)  AddHeaderDeclaration=on  Function1Type=when block is updated (default)  Fct1BlockIn=CPU_Load  FctReturnBlockOut=off  DataCollected="s.chksm={ '115614-Feb-2017 12:54:00'};s.File1=reshape({ '  void  ShowOff()','  void  PrintCount(unsigned int value)','  void  PrintCPU(double CPU_Load)','  void  PrintInteger(unsigned int CPU_Load)'},1,4);"  ORDERING=None  SampleTime=-1  S_INPUT=[0]  S_INPUT_Size="[0  0  0  0  0  0  0  0  0  0]"  S_OUTPUT=[]  S_OUTPUT_Size=[]  S_ListCustomDatatype=S.S_ListCustomDatatype={};  MCHP_CRC=1068656  MCHP_MASTERLINK=Explorer1632_LCD/Microchip Master  PinDigitalInput=[]  PinDigitalOutput=[]  PinAnalogInput=[]
  C Function Call4 : MCHP_Blockset/User Functions/C Function Call  ParseFilesChkbx=on  ListFunctions1=Custom Function  Function1=void PrintTemperature(double temp)  AddHeaderDeclaration=on  Function1Type=when block is updated (default)  Fct1BlockIn=temp  FctReturnBlockOut=off  DataCollected="s.chksm={ '148414-Feb-2017 17:33:09'};s.File1=reshape({ '  void  ShowOff()','  void  PrintMinutes(unsigned int value)','  void  PrintSeconds(unsigned int value)','  void  PrintCPU(double CPU_Load)','  void  PrintInteger(unsigned int CPU_Load)','  void  PrintTemperature(double temp)'},1,6);"  ORDERING=None  SampleTime=-1  S_INPUT=[0]  S_INPUT_Size="[0  0  0  0  0  0  0  0  0  0]"  S_OUTPUT=[]  S_OUTPUT_Size=[]  S_ListCustomDatatype=S.S_ListCustomDatatype={};  MCHP_CRC=1289936  MCHP_MASTERLINK=Explorer1632_LCD/Microchip Master  PinDigitalInput=[]  PinDigitalOutput=[]  PinAnalogInput=[]
  wires:
  In1/1 -> C Function Call2/1
  In2/1 -> C Function Call4/1
